simulink model "DatcomNew"  (R2017a)
settings: Solver=VariableStepAuto  StartTime=0.0  StopTime=10.0  RelTol=1e-3
undefined symbols (not defined in the file or in its folder): datcom, Newton, Raphson
libraries: aerolibutil x32, sharedutil x4, aerolibtransform2 x3, aerolibasang x3, aerolibadyn x1
(part 2 of 4)

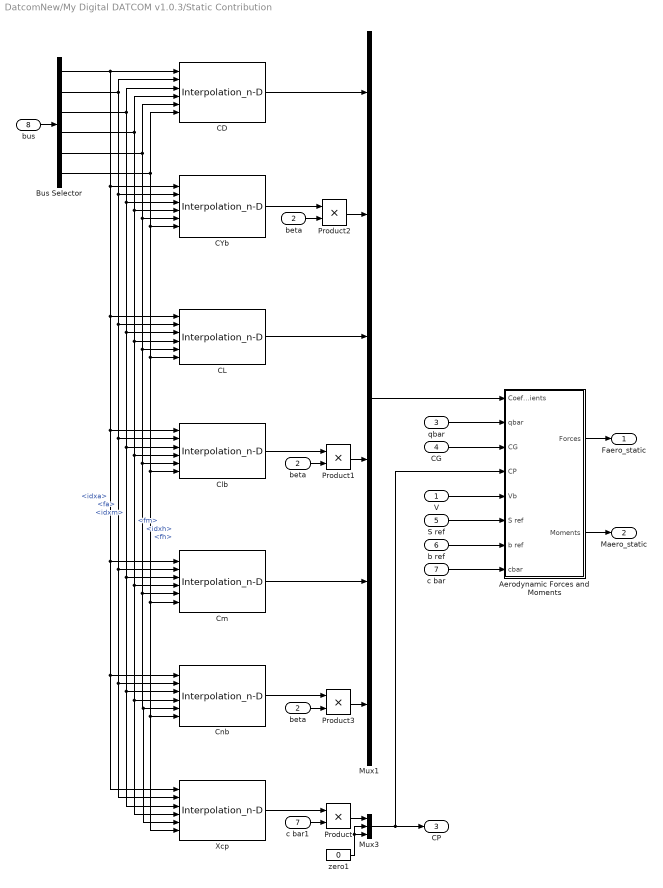
== system DatcomNew/My Digital DATCOM v1.0.3/Static Contribution ==
  "V " : Inport
  beta : Inport  Port=2
  qbar : Inport  Port=3
  CG : Inport  Port=4
  S ref : Inport  Port=5  Unit=m^2
  b ref : Inport  Port=6  Unit=m  PortDimensions=1
  c bar : Inport  Port=7  Unit=m  PortDimensions=1
  bus : Inport  Port=8
  " beta " : InportShadow  Port=2
  Aerodynamic Forces and Moments : Subsystem
  Bus Selector : BusSelector  OutputSignals=idxa,fa,idxm,fm,idxh,fh
  CD : Interpolation_n-D  NumberOfTableDimensions=3  Table=permute(datcom.cd,[1 2 3])  InterpMethod=Flat  ExtrapMethod=Clip  OutDataTypeStr=double
      settings: InputPortMap=u0,u1,u2,u3,u4,u5
  CL : Interpolation_n-D  NumberOfTableDimensions=3  Table=permute(datcom.cl,[1 2 3])  InterpMethod=Flat  ExtrapMethod=Clip  OutDataTypeStr=double
      settings: InputPortMap=u0,u1,u2,u3,u4,u5
  CYb : Interpolation_n-D  NumberOfTableDimensions=3  Table=permute(datcom.cyb,[1 2 3])  InterpMethod=Flat  ExtrapMethod=Clip  OutDataTypeStr=double
      settings: InputPortMap=u0,u1,u2,u3,u4,u5
  Clb : Interpolation_n-D  NumberOfTableDimensions=3  Table=permute(datcom.clb,[1 2 3])  InterpMethod=Flat  ExtrapMethod=Clip  OutDataTypeStr=double
      settings: InputPortMap=u0,u1,u2,u3,u4,u5
  Cm : Interpolation_n-D  NumberOfTableDimensions=3  Table=permute(datcom.cm,[1 2 3])  InterpMethod=Flat  ExtrapMethod=Clip  OutDataTypeStr=double
      settings: InputPortMap=u0,u1,u2,u3,u4,u5
  Cnb : Interpolation_n-D  NumberOfTableDimensions=3  Table=permute(datcom.cnb,[1 2 3])  InterpMethod=Flat  ExtrapMethod=Clip  OutDataTypeStr=double
      settings: InputPortMap=u0,u1,u2,u3,u4,u5
  Mux1 : Mux  Inputs=6
  Mux3 : Mux  Inputs=3
  Product : Product
  Product1 : Product  RndMeth=Zero
  Product2 : Product  RndMeth=Zero
  Product3 : Product  RndMeth=Zero
  Xcp : Interpolation_n-D  NumberOfTableDimensions=3  Table="permute(datcom.xcp,[1  2  3])"  OutDataTypeStr=double
      settings: InputPortMap=u0,u1,u2,u3,u4,u5
  "beta " : InportShadow  Port=2
  c bar1 : InportShadow  Port=7  Unit=m  PortDimensions=1
  zero1 : Constant  Value=0
  Faero_static : Outport
  Maero_static : Outport  Port=2
  "CP " : Outport  Port=3
  wires:
  c bar1/1 -> Product/2
  Product/1 -> Mux3/1
  zero1/1 -> Mux3/3, Mux3/2
  Xcp/1 -> Product/1
  c bar/1 -> Aerodynamic Forces and Moments/8(cbar)
  b ref/1 -> Aerodynamic Forces and Moments/7(b ref)
  S ref/1 -> Aerodynamic Forces and Moments/6(S ref)
  Mux3/1 -> Aerodynamic Forces and Moments/4(CP), "CP "/1
  CG/1 -> Aerodynamic Forces and Moments/3(CG)
  bus/1 -> Bus Selector/1
  Bus Selector/1 -> CD/1, CYb/1, Clb/1, Cnb/1, Xcp/1, Cm/1, CL/1  "<idxa>"
  Bus Selector/2 -> Cnb/2, Xcp/2, Cm/2, Clb/2, CL/2, CYb/2, CD/2  "<fa>"
  Bus Selector/3 -> Cnb/3, Xcp/3, Cm/3, Clb/3, CL/3, CYb/3, CD/3  "<idxm>"
  Bus Selector/4 -> Cnb/4, Xcp/4, Cm/4, Clb/4, CL/4, CYb/4, CD/4  "<fm>"
  Bus Selector/5 -> Cnb/5, Xcp/5, Cm/5, Clb/5, CL/5, CYb/5, CD/5  "<idxh>"
  Bus Selector/6 -> Cnb/6, Xcp/6, Cm/6, Clb/6, CL/6, CYb/6, CD/6  "<fh>"
  CD/1 -> Mux1/1
  CL/1 -> Mux1/3
  CYb/1 -> Product2/1
  beta/1 -> Product2/2
  Clb/1 -> Product1/1
  "beta "/1 -> Product1/2
  Product2/1 -> Mux1/2
  Product1/1 -> Mux1/4
  Cm/1 -> Mux1/5
  Cnb/1 -> Product3/1
  " beta "/1 -> Product3/2
  Product3/1 -> Mux1/6
  Mux1/1 -> Aerodynamic Forces and Moments/1(Coefficients)
  Aerodynamic Forces and Moments/1(Forces) -> Faero_static/1
  qbar/1 -> Aerodynamic Forces and Moments/2(qbar)
  Aerodynamic Forces and Moments/2(Moments) -> Maero_static/1
  "V "/1 -> Aerodynamic Forces and Moments/5(Vb)

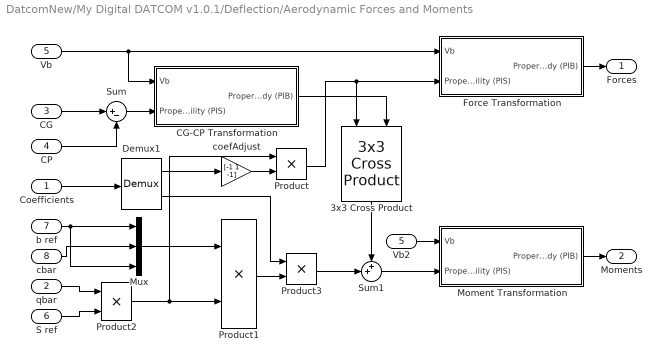
== system DatcomNew/My Digital DATCOM v1.0.1/Deflection/Aerodynamic Forces and Moments ==
  Coefficients : Inport
  qbar : Inport  Port=2  Unit=Pa
  CG : Inport  Port=3  Unit=m  PortDimensions=[3, 1]
  CP : Inport  Port=4  Unit=m  PortDimensions=[3,1]
  Vb : Inport  Port=5
  S ref : Inport  Port=6  Unit=m^2  PortDimensions=1
  b ref : Inport  Port=7  Unit=m  PortDimensions=1
  cbar : Inport  Port=8  Unit=m  PortDimensions=1
  3x3 Cross Product : aerolibutil/3x3 Cross Product
      settings: SourceProductName=Aerospace Blockset  SourceProductBaseCode=AE
  CG-CP Transformation : Subsystem
  Demux1 : Demux  Outputs=[3,3]
  Force Transformation : Subsystem
  Moment Transformation : Subsystem
  Mux : Mux  Inputs=3
  Product{,1..3} (4 alike) : Product  SaturateOnIntegerOverflow=on  InputSameDT=on  OutDataTypeStr=Inherit: Same as first input
  Sum : Sum  Inputs=|+-  SaturateOnIntegerOverflow=on
  Sum1 : Sum  Inputs=++|  SaturateOnIntegerOverflow=on  InputSameDT=on  OutDataTypeStr=Inherit: Same as first input
  Vb2 : InportShadow  Port=5
  coefAdjust : Gain  Gain="[-1  1 -1]"
  Forces : Outport  Unit=N
  Moments : Outport  Port=2  Unit=N
  wires:
  Vb/1 -> CG-CP Transformation/1(Vb), Force Transformation/1(Vb)
  CG-CP Transformation/1(Property-In-Body (PIB)) -> 3x3 Cross Product/2
  Sum/1 -> CG-CP Transformation/2(Property-In-Stability (PIS))
  CP/1 -> Sum/2
  CG/1 -> Sum/1
  coefAdjust/1 -> Product/2
  Moment Transformation/1(Property-In-Body (PIB)) -> Moments/1
  Force Transformation/1(Property-In-Body (PIB)) -> Forces/1
  Product/1 -> 3x3 Cross Product/1, Force Transformation/2(Property-In-Stability (PIS))
  Demux1/1 -> coefAdjust/1
  Product3/1 -> Sum1/2
  Product2/1 -> Product/1, Product1/2
  qbar/1 -> Product2/1
  Demux1/2 -> Product3/1
  Coefficients/1 -> Demux1/1
  Product1/1 -> Product3/2
  3x3 Cross Product/1 -> Sum1/1
  cbar/1 -> Mux/2
  b ref/1 -> Mux/1, Mux/3
  Mux/1 -> Product1/1
  S ref/1 -> Product2/2
  Sum1/1 -> Moment Transformation/2(Property-In-Stability (PIS))
  Vb2/1 -> Moment Transformation/1(Vb)

== system DatcomNew/My Digital DATCOM v1.0.1/Deflection/Delta Coefficients ==
  bus : Inport
  Aileron Deflaction : Subsystem
  Elevator Deflaction : Subsystem
  Flap Deflaction : Subsystem
  Sum : Sum  Inputs=+++
  delCoeff : Outport
  wires:
  bus/1 -> Flap Deflaction/1(bus), Aileron Deflaction/1(bus), Elevator Deflaction/1(bus)
  Elevator Deflaction/1(delCoeff_e) -> Sum/2
  Flap Deflaction/1(delCoeff_f) -> Sum/1
  Aileron Deflaction/1(delCoeff_a) -> Sum/3
  Sum/1 -> delCoeff/1

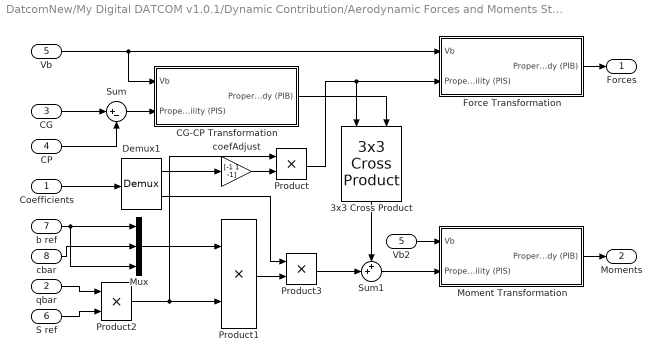
== system DatcomNew/My Digital DATCOM v1.0.1/Dynamic Contribution/Aerodynamic Forces and Moments Stability Axis ==
  Coefficients : Inport
  qbar : Inport  Port=2  Unit=Pa
  CG : Inport  Port=3  Unit=m  PortDimensions=[3, 1]
  CP : Inport  Port=4  Unit=m  PortDimensions=[3,1]
  Vb : Inport  Port=5
  S ref : Inport  Port=6  Unit=m^2  PortDimensions=1
  b ref : Inport  Port=7  Unit=m  PortDimensions=1
  cbar : Inport  Port=8  Unit=m  PortDimensions=1
  3x3 Cross Product : aerolibutil/3x3 Cross Product
      settings: SourceProductName=Aerospace Blockset  SourceProductBaseCode=AE
  CG-CP Transformation : Subsystem
  Demux1 : Demux  Outputs=[3,3]
  Force Transformation : Subsystem
  Moment Transformation : Subsystem
  Mux : Mux  Inputs=3
  Product{,1..3} (4 alike) : Product  SaturateOnIntegerOverflow=on  InputSameDT=on  OutDataTypeStr=Inherit: Same as first input
  Sum : Sum  Inputs=|+-  SaturateOnIntegerOverflow=on
  Sum1 : Sum  Inputs=++|  SaturateOnIntegerOverflow=on  InputSameDT=on  OutDataTypeStr=Inherit: Same as first input
  Vb2 : InportShadow  Port=5
  coefAdjust : Gain  Gain="[-1  1 -1]"
  Forces : Outport  Unit=N
  Moments : Outport  Port=2  Unit=N*m
  wires:
  Vb/1 -> CG-CP Transformation/1(Vb), Force Transformation/1(Vb)
  CG-CP Transformation/1(Property-In-Body (PIB)) -> 3x3 Cross Product/2
  Sum/1 -> CG-CP Transformation/2(Property-In-Stability (PIS))
  CP/1 -> Sum/2
  CG/1 -> Sum/1
  coefAdjust/1 -> Product/2
  Moment Transformation/1(Property-In-Body (PIB)) -> Moments/1
  Force Transformation/1(Property-In-Body (PIB)) -> Forces/1
  Product/1 -> 3x3 Cross Product/1, Force Transformation/2(Property-In-Stability (PIS))
  Demux1/1 -> coefAdjust/1
  Product3/1 -> Sum1/2
  Product2/1 -> Product/1, Product1/2
  qbar/1 -> Product2/1
  Demux1/2 -> Product3/1
  Coefficients/1 -> Demux1/1
  Product1/1 -> Product3/2
  3x3 Cross Product/1 -> Sum1/1
  cbar/1 -> Mux/2
  b ref/1 -> Mux/1, Mux/3
  Mux/1 -> Product1/1
  S ref/1 -> Product2/2
  Sum1/1 -> Moment Transformation/2(Property-In-Stability (PIS))
  Vb2/1 -> Moment Transformation/1(Vb)

== system DatcomNew/My Digital DATCOM v1.0.1/Dynamic Contribution/Incidence, Sideslip, & Airspeed1 ==
  Vb : Inport  Unit=m/s
  Airspeed : Sqrt  AlgorithmType=Newton-Raphson  SaturateOnIntegerOverflow=on
  Dot Product : DotProduct  InputSameDT=on  OutDataTypeStr=Inherit: Inherit via internal rule
  Incidence : Trigonometry  Operator=atan2
  Product : Product  Inputs=*/  SaturateOnIntegerOverflow=on  OutDataTypeStr=Inherit: Same as first input
  Selector : Selector  InputPortWidth=3  IndexOptions=Index vector (dialog)  Indices=[2]  OutputSizes=1
  Selector1 : Selector  InputPortWidth=3  IndexOptions=Index vector (dialog)  Indices=[3]  OutputSizes=1
  Selector2 : Selector  InputPortWidth=3  IndexOptions=Index vector (dialog)  Indices=[1]  OutputSizes=1
  Sideslip : Trigonometry  Operator=asin
  Alpha : Outport  Unit=rad  InitialOutput=0
  Beta : Outport  Port=2  Unit=rad  InitialOutput=0
  V : Outport  Port=3  Unit=m/s  InitialOutput=0
  wires:
  Product/1 -> Sideslip/1
  Selector1/1 -> Incidence/1
  Selector2/1 -> Incidence/2
  Dot Product/1 -> Airspeed/1
  Airspeed/1 -> Product/2, V/1
  Incidence/1 -> Alpha/1
  Vb/1 -> Selector1/1, Selector2/1, Selector/1, Dot Product/1, Dot Product/2
  Sideslip/1 -> Beta/1
  Selector/1 -> Product/1

== system DatcomNew/My Digital DATCOM v1.0.1/Dynamic Contribution/Stability Angular Rates ==
  alpha beta : Inport  Unit=rad
  alphadot betadot : Inport  Port=2  Unit=rad/s
  p,q,r : Inport  Port=3  Unit=rad/s
  Demux : Demux  Outputs=2
  Direction Cosine Matrix Body to Wind : aerolibtransform2/Direction Cosine Matrix Body to Wind
      settings: SourceProductName=Aerospace Blockset  SourceProductBaseCode=AE
  Disallow CGS : UnitConfiguration  UnitSystemsStr=English,SI,SI (extended)  AllowAllUnitSystems=off
  Mux : Mux  Inputs=3
  Product : Product  RndMeth=Zero
  Product1 : Product  Multiplication=Matrix(*)  SaturateOnIntegerOverflow=on  InputSameDT=on  OutDataTypeStr=Inherit: Same as first input
  Product2 : Product  RndMeth=Zero
  SinCos : Trigonometry  Operator=sincos
  Subsystem : aerolibasang/Wind Angular Rates/Subsystem
      settings: SourceProductName=Aerospace Blockset  SourceProductBaseCode=AE
  Sum : Sum  Inputs=|++
  Unary Minus : UnaryMinus
  Unary Minus1 : UnaryMinus
  p,q,r wind : Outport  Unit=rad/s  InitialOutput=0
  wires:
  Unary Minus/1 -> Mux/2
  Unary Minus1/1 -> Mux/1
  Product2/1 -> Mux/3
  Product/1 -> Unary Minus1/1
  Demux/1 -> Unary Minus/1
  Demux/2 -> Product/1, Product2/1
  alphadot betadot/1 -> Demux/1
  p,q,r/1 -> Sum/2
  Mux/1 -> Sum/1
  Product1/1 -> p,q,r wind/1
  Sum/1 -> Product1/2
  Direction Cosine Matrix Body to Wind/1 -> Product1/1
  SinCos/2 -> Product2/2
  SinCos/1 -> Product/2
  Subsystem/1 -> SinCos/1
  alpha beta/1 -> Subsystem/1, Direction Cosine Matrix Body to Wind/1

== system DatcomNew/My Digital DATCOM v1.0.1/Static Contribution/Aerodynamic Forces and Moments ==
  Coefficients : Inport
  qbar : Inport  Port=2  Unit=Pa
  CG : Inport  Port=3  Unit=m  PortDimensions=[3, 1]
  CP : Inport  Port=4  Unit=m  PortDimensions=[3,1]
  Vb : Inport  Port=5
  S ref : Inport  Port=6  Unit=m^2  PortDimensions=1
  b ref : Inport  Port=7  Unit=m  PortDimensions=1
  cbar : Inport  Port=8  Unit=m  PortDimensions=1
  3x3 Cross Product : aerolibutil/3x3 Cross Product
      settings: SourceProductName=Aerospace Blockset  SourceProductBaseCode=AE
  CG-CP Transformation : Subsystem
  Demux1 : Demux  Outputs=[3,3]
  Force Transformation : Subsystem
  Moment Transformation : Subsystem
  Mux : Mux  Inputs=3
  Product{,1..3} (4 alike) : Product  SaturateOnIntegerOverflow=on  InputSameDT=on  OutDataTypeStr=Inherit: Same as first input
  Sum : Sum  Inputs=|+-  SaturateOnIntegerOverflow=on
  Sum1 : Sum  Inputs=++|  SaturateOnIntegerOverflow=on  InputSameDT=on  OutDataTypeStr=Inherit: Same as first input
  Vb2 : InportShadow  Port=5
  coefAdjust : Gain  Gain="[-1  1 -1]"
  Forces : Outport  Unit=N
  Moments : Outport  Port=2  Unit=N*m
  wires:
  Vb/1 -> CG-CP Transformation/1(Vb), Force Transformation/1(Vb)
  CG-CP Transformation/1(Property-In-Body (PIB)) -> 3x3 Cross Product/2
  Sum/1 -> CG-CP Transformation/2(Property-In-Stability (PIS))
  CP/1 -> Sum/2
  CG/1 -> Sum/1
  coefAdjust/1 -> Product/2
  Moment Transformation/1(Property-In-Body (PIB)) -> Moments/1
  Force Transformation/1(Property-In-Body (PIB)) -> Forces/1
  Product/1 -> 3x3 Cross Product/1, Force Transformation/2(Property-In-Stability (PIS))
  Demux1/1 -> coefAdjust/1
  Product3/1 -> Sum1/2
  Product2/1 -> Product/1, Product1/2
  qbar/1 -> Product2/1
  Demux1/2 -> Product3/1
  Coefficients/1 -> Demux1/1
  Product1/1 -> Product3/2
  3x3 Cross Product/1 -> Sum1/1
  cbar/1 -> Mux/2
  b ref/1 -> Mux/1, Mux/3
  Mux/1 -> Product1/1
  S ref/1 -> Product2/2
  Sum1/1 -> Moment Transformation/2(Property-In-Stability (PIS))
  Vb2/1 -> Moment Transformation/1(Vb)

== system DatcomNew/My Digital DATCOM v1.0.2/Deflection/Aerodynamic Forces and Moments ==
  Coefficients : Inport
  qbar : Inport  Port=2  Unit=Pa
  CG : Inport  Port=3  Unit=m  PortDimensions=[3, 1]
  CP : Inport  Port=4  Unit=m  PortDimensions=[3,1]
  Vb : Inport  Port=5
  S ref : Inport  Port=6  Unit=m^2  PortDimensions=1
  b ref : Inport  Port=7  Unit=m  PortDimensions=1
  cbar : Inport  Port=8  Unit=m  PortDimensions=1
  3x3 Cross Product : aerolibutil/3x3 Cross Product
      settings: SourceProductName=Aerospace Blockset  SourceProductBaseCode=AE
  CG-CP Transformation : Subsystem
  Demux1 : Demux  Outputs=[3,3]
  Force Transformation : Subsystem
  Moment Transformation : Subsystem
  Mux : Mux  Inputs=3
  Product{,1..3} (4 alike) : Product  SaturateOnIntegerOverflow=on  InputSameDT=on  OutDataTypeStr=Inherit: Same as first input
  Sum : Sum  Inputs=|+-  SaturateOnIntegerOverflow=on
  Sum1 : Sum  Inputs=++|  SaturateOnIntegerOverflow=on  InputSameDT=on  OutDataTypeStr=Inherit: Same as first input
  Vb2 : InportShadow  Port=5
  coefAdjust : Gain  Gain="[-1  1 -1]"
  Forces : Outport  Unit=N
  Moments : Outport  Port=2  Unit=N
  wires:
  Vb2/1 -> Moment Transformation/1(Vb)
  Sum1/1 -> Moment Transformation/2(Property-In-Stability (PIS))
  S ref/1 -> Product2/2
  Mux/1 -> Product1/1
  b ref/1 -> Mux/3, Mux/1
  cbar/1 -> Mux/2
  3x3 Cross Product/1 -> Sum1/1
  Product1/1 -> Product3/2
  Coefficients/1 -> Demux1/1
  Demux1/2 -> Product3/1
  qbar/1 -> Product2/1
  Product2/1 -> Product1/2, Product/1
  Product3/1 -> Sum1/2
  Demux1/1 -> coefAdjust/1
  Product/1 -> Force Transformation/2(Property-In-Stability (PIS)), 3x3 Cross Product/1
  Force Transformation/1(Property-In-Body (PIB)) -> Forces/1
  Moment Transformation/1(Property-In-Body (PIB)) -> Moments/1
  coefAdjust/1 -> Product/2
  CG/1 -> Sum/1
  CP/1 -> Sum/2
  Sum/1 -> CG-CP Transformation/2(Property-In-Stability (PIS))
  CG-CP Transformation/1(Property-In-Body (PIB)) -> 3x3 Cross Product/2
  Vb/1 -> Force Transformation/1(Vb), CG-CP Transformation/1(Vb)

== system DatcomNew/My Digital DATCOM v1.0.2/Deflection/Delta Coefficients ==
  bus : Inport
  Aileron Deflaction : Subsystem
  Elevator Deflaction : Subsystem
  Flap Deflaction : Subsystem
  Sum : Sum  Inputs=+++
  delCoeff : Outport
  wires:
  Sum/1 -> delCoeff/1
  Aileron Deflaction/1(delCoeff_a) -> Sum/3
  Flap Deflaction/1(delCoeff_f) -> Sum/1
  Elevator Deflaction/1(delCoeff_e) -> Sum/2
  bus/1 -> Elevator Deflaction/1(bus), Aileron Deflaction/1(bus), Flap Deflaction/1(bus)

== system DatcomNew/My Digital DATCOM v1.0.2/Dynamic Contribution/Aerodynamic Forces and Moments Stability Axis ==
  Coefficients : Inport
  qbar : Inport  Port=2  Unit=Pa
  CG : Inport  Port=3  Unit=m  PortDimensions=[3, 1]
  CP : Inport  Port=4  Unit=m  PortDimensions=[3,1]
  Vb : Inport  Port=5
  S ref : Inport  Port=6  Unit=m^2  PortDimensions=1
  b ref : Inport  Port=7  Unit=m  PortDimensions=1
  cbar : Inport  Port=8  Unit=m  PortDimensions=1
  3x3 Cross Product : aerolibutil/3x3 Cross Product
      settings: SourceProductName=Aerospace Blockset  SourceProductBaseCode=AE
  CG-CP Transformation : Subsystem
  Demux1 : Demux  Outputs=[3,3]
  Force Transformation : Subsystem
  Moment Transformation : Subsystem
  Mux : Mux  Inputs=3
  Product{,1..3} (4 alike) : Product  SaturateOnIntegerOverflow=on  InputSameDT=on  OutDataTypeStr=Inherit: Same as first input
  Sum : Sum  Inputs=|+-  SaturateOnIntegerOverflow=on
  Sum1 : Sum  Inputs=++|  SaturateOnIntegerOverflow=on  InputSameDT=on  OutDataTypeStr=Inherit: Same as first input
  Vb2 : InportShadow  Port=5
  coefAdjust : Gain  Gain="[-1  1 -1]"
  Forces : Outport  Unit=N
  Moments : Outport  Port=2  Unit=N*m
  wires:
  Vb2/1 -> Moment Transformation/1(Vb)
  Sum1/1 -> Moment Transformation/2(Property-In-Stability (PIS))
  S ref/1 -> Product2/2
  Mux/1 -> Product1/1
  b ref/1 -> Mux/3, Mux/1
  cbar/1 -> Mux/2
  3x3 Cross Product/1 -> Sum1/1
  Product1/1 -> Product3/2
  Coefficients/1 -> Demux1/1
  Demux1/2 -> Product3/1
  qbar/1 -> Product2/1
  Product2/1 -> Product1/2, Product/1
  Product3/1 -> Sum1/2
  Demux1/1 -> coefAdjust/1
  Product/1 -> Force Transformation/2(Property-In-Stability (PIS)), 3x3 Cross Product/1
  Force Transformation/1(Property-In-Body (PIB)) -> Forces/1
  Moment Transformation/1(Property-In-Body (PIB)) -> Moments/1
  coefAdjust/1 -> Product/2
  CG/1 -> Sum/1
  CP/1 -> Sum/2
  Sum/1 -> CG-CP Transformation/2(Property-In-Stability (PIS))
  CG-CP Transformation/1(Property-In-Body (PIB)) -> 3x3 Cross Product/2
  Vb/1 -> Force Transformation/1(Vb), CG-CP Transformation/1(Vb)

== system DatcomNew/My Digital DATCOM v1.0.2/Dynamic Contribution/Incidence, Sideslip, & Airspeed1 ==
  Vb : Inport  Unit=m/s
  Airspeed : Sqrt  AlgorithmType=Newton-Raphson  SaturateOnIntegerOverflow=on
  Dot Product : DotProduct  InputSameDT=on  OutDataTypeStr=Inherit: Inherit via internal rule
  Incidence : Trigonometry  Operator=atan2
  Product : Product  Inputs=*/  SaturateOnIntegerOverflow=on  OutDataTypeStr=Inherit: Same as first input
  Selector : Selector  InputPortWidth=3  IndexOptions=Index vector (dialog)  Indices=[2]  OutputSizes=1
  Selector1 : Selector  InputPortWidth=3  IndexOptions=Index vector (dialog)  Indices=[3]  OutputSizes=1
  Selector2 : Selector  InputPortWidth=3  IndexOptions=Index vector (dialog)  Indices=[1]  OutputSizes=1
  Sideslip : Trigonometry  Operator=asin
  Alpha : Outport  Unit=rad  InitialOutput=0
  Beta : Outport  Port=2  Unit=rad  InitialOutput=0
  V : Outport  Port=3  Unit=m/s  InitialOutput=0
  wires:
  Selector/1 -> Product/1
  Sideslip/1 -> Beta/1
  Vb/1 -> Dot Product/2, Dot Product/1, Selector/1, Selector2/1, Selector1/1
  Incidence/1 -> Alpha/1
  Airspeed/1 -> V/1, Product/2
  Dot Product/1 -> Airspeed/1
  Selector2/1 -> Incidence/2
  Selector1/1 -> Incidence/1
  Product/1 -> Sideslip/1

== system DatcomNew/My Digital DATCOM v1.0.2/Dynamic Contribution/Stability Angular Rates ==
  alpha beta : Inport  Unit=rad
  alphadot betadot : Inport  Port=2  Unit=rad/s
  p,q,r : Inport  Port=3  Unit=rad/s
  Demux : Demux  Outputs=2
  Direction Cosine Matrix Body to Wind : aerolibtransform2/Direction Cosine Matrix Body to Wind
      settings: SourceProductName=Aerospace Blockset  SourceProductBaseCode=AE
  Disallow CGS : UnitConfiguration  UnitSystemsStr=English,SI,SI (extended)  AllowAllUnitSystems=off
  Mux : Mux  Inputs=3
  Product : Product  RndMeth=Zero
  Product1 : Product  Multiplication=Matrix(*)  SaturateOnIntegerOverflow=on  InputSameDT=on  OutDataTypeStr=Inherit: Same as first input
  Product2 : Product  RndMeth=Zero
  SinCos : Trigonometry  Operator=sincos
  Subsystem : aerolibasang/Wind Angular Rates/Subsystem
      settings: SourceProductName=Aerospace Blockset  SourceProductBaseCode=AE
  Sum : Sum  Inputs=|++
  Unary Minus : UnaryMinus
  Unary Minus1 : UnaryMinus
  p,q,r wind : Outport  Unit=rad/s  InitialOutput=0
  wires:
  alpha beta/1 -> Direction Cosine Matrix Body to Wind/1, Subsystem/1
  Subsystem/1 -> SinCos/1
  SinCos/1 -> Product/2
  SinCos/2 -> Product2/2
  Direction Cosine Matrix Body to Wind/1 -> Product1/1
  Sum/1 -> Product1/2
  Product1/1 -> p,q,r wind/1
  Mux/1 -> Sum/1
  p,q,r/1 -> Sum/2
  alphadot betadot/1 -> Demux/1
  Demux/2 -> Product2/1, Product/1
  Demux/1 -> Unary Minus/1
  Product/1 -> Unary Minus1/1
  Product2/1 -> Mux/3
  Unary Minus1/1 -> Mux/1
  Unary Minus/1 -> Mux/2

== system DatcomNew/My Digital DATCOM v1.0.2/Static Contribution/Aerodynamic Forces and Moments ==
  Coefficients : Inport
  qbar : Inport  Port=2  Unit=Pa
  CG : Inport  Port=3  Unit=m  PortDimensions=[3, 1]
  CP : Inport  Port=4  Unit=m  PortDimensions=[3,1]
  Vb : Inport  Port=5
  S ref : Inport  Port=6  Unit=m^2  PortDimensions=1
  b ref : Inport  Port=7  Unit=m  PortDimensions=1
  cbar : Inport  Port=8  Unit=m  PortDimensions=1
  3x3 Cross Product : aerolibutil/3x3 Cross Product
      settings: SourceProductName=Aerospace Blockset  SourceProductBaseCode=AE
  CG-CP Transformation : Subsystem
  Demux1 : Demux  Outputs=[3,3]
  Force Transformation : Subsystem
  Moment Transformation : Subsystem
  Mux : Mux  Inputs=3
  Product{,1..3} (4 alike) : Product  SaturateOnIntegerOverflow=on  InputSameDT=on  OutDataTypeStr=Inherit: Same as first input
  Sum : Sum  Inputs=|+-  SaturateOnIntegerOverflow=on
  Sum1 : Sum  Inputs=++|  SaturateOnIntegerOverflow=on  InputSameDT=on  OutDataTypeStr=Inherit: Same as first input
  Vb2 : InportShadow  Port=5
  coefAdjust : Gain  Gain="[-1  1 -1]"
  Forces : Outport  Unit=N
  Moments : Outport  Port=2  Unit=N*m
  wires:
  Vb2/1 -> Moment Transformation/1(Vb)
  Sum1/1 -> Moment Transformation/2(Property-In-Stability (PIS))
  S ref/1 -> Product2/2
  Mux/1 -> Product1/1
  b ref/1 -> Mux/3, Mux/1
  cbar/1 -> Mux/2
  3x3 Cross Product/1 -> Sum1/1
  Product1/1 -> Product3/2
  Coefficients/1 -> Demux1/1
  Demux1/2 -> Product3/1
  qbar/1 -> Product2/1
  Product2/1 -> Product1/2, Product/1
  Product3/1 -> Sum1/2
  Demux1/1 -> coefAdjust/1
  Product/1 -> Force Transformation/2(Property-In-Stability (PIS)), 3x3 Cross Product/1
  Force Transformation/1(Property-In-Body (PIB)) -> Forces/1
  Moment Transformation/1(Property-In-Body (PIB)) -> Moments/1
  coefAdjust/1 -> Product/2
  CG/1 -> Sum/1
  CP/1 -> Sum/2
  Sum/1 -> CG-CP Transformation/2(Property-In-Stability (PIS))
  CG-CP Transformation/1(Property-In-Body (PIB)) -> 3x3 Cross Product/2
  Vb/1 -> Force Transformation/1(Vb), CG-CP Transformation/1(Vb)

== system DatcomNew/My Digital DATCOM v1.0.3/Deflection/Aerodynamic Forces and Moments ==
  Coefficients : Inport
  qbar : Inport  Port=2  Unit=Pa
  CG : Inport  Port=3  Unit=m  PortDimensions=[3, 1]
  CP : Inport  Port=4  Unit=m  PortDimensions=[3,1]
  Vb : Inport  Port=5
  S ref : Inport  Port=6  Unit=m^2  PortDimensions=1
  b ref : Inport  Port=7  Unit=m  PortDimensions=1
  cbar : Inport  Port=8  Unit=m  PortDimensions=1
  3x3 Cross Product : aerolibutil/3x3 Cross Product
      settings: SourceProductName=Aerospace Blockset  SourceProductBaseCode=AE
  CG-CP Transformation : Subsystem
  Demux1 : Demux  Outputs=[3,3]
  Force Transformation : Subsystem
  Moment Transformation : Subsystem
  Mux : Mux  Inputs=3
  Product{,1..3} (4 alike) : Product  SaturateOnIntegerOverflow=on  InputSameDT=on  OutDataTypeStr=Inherit: Same as first input
  Sum : Sum  Inputs=|+-  SaturateOnIntegerOverflow=on
  Sum1 : Sum  Inputs=++|  SaturateOnIntegerOverflow=on  InputSameDT=on  OutDataTypeStr=Inherit: Same as first input
  Vb2 : InportShadow  Port=5
  coefAdjust : Gain  Gain="[-1  1 -1]"
  Forces : Outport  Unit=N
  Moments : Outport  Port=2  Unit=N
  wires:
  Vb2/1 -> Moment Transformation/1(Vb)
  Sum1/1 -> Moment Transformation/2(Property-In-Stability (PIS))
  S ref/1 -> Product2/2
  Mux/1 -> Product1/1
  b ref/1 -> Mux/3, Mux/1
  cbar/1 -> Mux/2
  3x3 Cross Product/1 -> Sum1/1
  Product1/1 -> Product3/2
  Coefficients/1 -> Demux1/1
  Demux1/2 -> Product3/1
  qbar/1 -> Product2/1
  Product2/1 -> Product1/2, Product/1
  Product3/1 -> Sum1/2
  Demux1/1 -> coefAdjust/1
  Product/1 -> Force Transformation/2(Property-In-Stability (PIS)), 3x3 Cross Product/1
  Force Transformation/1(Property-In-Body (PIB)) -> Forces/1
  Moment Transformation/1(Property-In-Body (PIB)) -> Moments/1
  coefAdjust/1 -> Product/2
  CG/1 -> Sum/1
  CP/1 -> Sum/2
  Sum/1 -> CG-CP Transformation/2(Property-In-Stability (PIS))
  CG-CP Transformation/1(Property-In-Body (PIB)) -> 3x3 Cross Product/2
  Vb/1 -> Force Transformation/1(Vb), CG-CP Transformation/1(Vb)

== system DatcomNew/My Digital DATCOM v1.0.3/Deflection/Delta Coefficients ==
  bus : Inport
  Aileron Deflaction : Subsystem
  Elevator Deflaction : Subsystem
  Flap Deflaction : Subsystem
  Sum : Sum  Inputs=+++
  delCoeff : Outport
  wires:
  Sum/1 -> delCoeff/1
  Aileron Deflaction/1(delCoeff_a) -> Sum/3
  Flap Deflaction/1(delCoeff_f) -> Sum/1
  Elevator Deflaction/1(delCoeff_e) -> Sum/2
  bus/1 -> Elevator Deflaction/1(bus), Aileron Deflaction/1(bus), Flap Deflaction/1(bus)

== system DatcomNew/My Digital DATCOM v1.0.3/Dynamic Contribution/Aerodynamic Forces and Moments Stability Axis ==
  Coefficients : Inport
  qbar : Inport  Port=2  Unit=Pa
  CG : Inport  Port=3  Unit=m  PortDimensions=[3, 1]
  CP : Inport  Port=4  Unit=m  PortDimensions=[3,1]
  Vb : Inport  Port=5
  S ref : Inport  Port=6  Unit=m^2  PortDimensions=1
  b ref : Inport  Port=7  Unit=m  PortDimensions=1
  cbar : Inport  Port=8  Unit=m  PortDimensions=1
  3x3 Cross Product : sharedutil/3x3 Cross Product
  CG-CP Transformation : Subsystem
  Demux1 : Demux  Outputs=[3,3]
  Force Transformation : Subsystem
  Moment Transformation : Subsystem
  Mux : Mux  Inputs=3
  Product{,1..3} (4 alike) : Product  SaturateOnIntegerOverflow=on  InputSameDT=on  OutDataTypeStr=Inherit: Same as first input
  Sum : Sum  Inputs=|+-  SaturateOnIntegerOverflow=on
  Sum1 : Sum  Inputs=++|  SaturateOnIntegerOverflow=on  InputSameDT=on  OutDataTypeStr=Inherit: Same as first input
  Vb2 : InportShadow  Port=5
  coefAdjust : Gain  Gain="[-1  1 -1]"
  Forces : Outport  Unit=N
  Moments : Outport  Port=2  Unit=N*m
  wires:
  Vb2/1 -> Moment Transformation/1(Vb)
  Sum1/1 -> Moment Transformation/2(Property-In-Stability (PIS))
  S ref/1 -> Product2/2
  Mux/1 -> Product1/1
  b ref/1 -> Mux/3, Mux/1
  cbar/1 -> Mux/2
  3x3 Cross Product/1 -> Sum1/1
  Product1/1 -> Product3/2
  Coefficients/1 -> Demux1/1
  Demux1/2 -> Product3/1
  qbar/1 -> Product2/1
  Product2/1 -> Product1/2, Product/1
  Product3/1 -> Sum1/2
  Demux1/1 -> coefAdjust/1
  Product/1 -> Force Transformation/2(Property-In-Stability (PIS)), 3x3 Cross Product/1
  Force Transformation/1(Property-In-Body (PIB)) -> Forces/1
  Moment Transformation/1(Property-In-Body (PIB)) -> Moments/1
  coefAdjust/1 -> Product/2
  CG/1 -> Sum/1
  CP/1 -> Sum/2
  Sum/1 -> CG-CP Transformation/2(Property-In-Stability (PIS))
  CG-CP Transformation/1(Property-In-Body (PIB)) -> 3x3 Cross Product/2
  Vb/1 -> Force Transformation/1(Vb), CG-CP Transformation/1(Vb)

== system DatcomNew/My Digital DATCOM v1.0.3/Dynamic Contribution/Incidence, Sideslip, & Airspeed1 ==
  Vb : Inport  Unit=m/s
  Airspeed : Sqrt  AlgorithmType=Newton-Raphson  SaturateOnIntegerOverflow=on
  Dot Product : DotProduct  InputSameDT=on  OutDataTypeStr=Inherit: Inherit via internal rule
  Incidence : Trigonometry  Operator=atan2
  Product : Product  Inputs=*/  SaturateOnIntegerOverflow=on  OutDataTypeStr=Inherit: Same as first input
  Selector : Selector  InputPortWidth=3  IndexOptions=Index vector (dialog)  Indices=[2]  OutputSizes=1
  Selector1 : Selector  InputPortWidth=3  IndexOptions=Index vector (dialog)  Indices=[3]  OutputSizes=1
  Selector2 : Selector  InputPortWidth=3  IndexOptions=Index vector (dialog)  Indices=[1]  OutputSizes=1
  Sideslip : Trigonometry  Operator=asin
  Alpha : Outport  Unit=rad  InitialOutput=0
  Beta : Outport  Port=2  Unit=rad  InitialOutput=0
  V : Outport  Port=3  Unit=m/s  InitialOutput=0
  wires:
  Selector/1 -> Product/1
  Sideslip/1 -> Beta/1
  Vb/1 -> Dot Product/2, Dot Product/1, Selector/1, Selector2/1, Selector1/1
  Incidence/1 -> Alpha/1
  Airspeed/1 -> V/1, Product/2
  Dot Product/1 -> Airspeed/1
  Selector2/1 -> Incidence/2
  Selector1/1 -> Incidence/1
  Product/1 -> Sideslip/1

== system DatcomNew/My Digital DATCOM v1.0.3/Dynamic Contribution/Stability Angular Rates ==
  alpha beta : Inport  Unit=rad
  alphadot betadot : Inport  Port=2  Unit=rad/s
  p,q,r : Inport  Port=3  Unit=rad/s
  Demux : Demux  Outputs=2
  Direction Cosine Matrix Body to Wind : aerolibtransform2/Direction Cosine Matrix Body to Wind
      settings: SourceProductName=Aerospace Blockset  SourceProductBaseCode=AE
  Disallow CGS : UnitConfiguration  UnitSystemsStr=English,SI,SI (extended)  AllowAllUnitSystems=off
  Mux : Mux  Inputs=3
  Product : Product  RndMeth=Zero
  Product1 : Product  Multiplication=Matrix(*)  SaturateOnIntegerOverflow=on  InputSameDT=on  OutDataTypeStr=Inherit: Same as first input
  Product2 : Product  RndMeth=Zero
  SinCos : Trigonometry  Operator=sincos
  Subsystem : aerolibasang/Wind Angular Rates/Subsystem
      settings: SourceProductName=Aerospace Blockset  SourceProductBaseCode=AE
  Sum : Sum  Inputs=|++
  Unary Minus : UnaryMinus
  Unary Minus1 : UnaryMinus
  p,q,r wind : Outport  Unit=rad/s  InitialOutput=0
  wires:
  alpha beta/1 -> Direction Cosine Matrix Body to Wind/1, Subsystem/1
  Subsystem/1 -> SinCos/1
  SinCos/1 -> Product/2
  SinCos/2 -> Product2/2
  Direction Cosine Matrix Body to Wind/1 -> Product1/1
  Sum/1 -> Product1/2
  Product1/1 -> p,q,r wind/1
  Mux/1 -> Sum/1
  p,q,r/1 -> Sum/2
  alphadot betadot/1 -> Demux/1
  Demux/2 -> Product2/1, Product/1
  Demux/1 -> Unary Minus/1
  Product/1 -> Unary Minus1/1
  Product2/1 -> Mux/3
  Unary Minus1/1 -> Mux/1
  Unary Minus/1 -> Mux/2

== system DatcomNew/My Digital DATCOM v1.0.3/Static Contribution/Aerodynamic Forces and Moments ==
  Coefficients : Inport
  qbar : Inport  Port=2  Unit=Pa
  CG : Inport  Port=3  Unit=m  PortDimensions=[3, 1]
  CP : Inport  Port=4  Unit=m  PortDimensions=[3,1]
  Vb : Inport  Port=5
  S ref : Inport  Port=6  Unit=m^2  PortDimensions=1
  b ref : Inport  Port=7  Unit=m  PortDimensions=1
  cbar : Inport  Port=8  Unit=m  PortDimensions=1
  3x3 Cross Product : aerolibutil/3x3 Cross Product
      settings: SourceProductName=Aerospace Blockset  SourceProductBaseCode=AE
  CG-CP Transformation : Subsystem
  Demux1 : Demux  Outputs=[3,3]
  Force Transformation : Subsystem
  Moment Transformation : Subsystem
  Mux : Mux  Inputs=3
  Product{,1..3} (4 alike) : Product  SaturateOnIntegerOverflow=on  InputSameDT=on  OutDataTypeStr=Inherit: Same as first input
  Sum : Sum  Inputs=|+-  SaturateOnIntegerOverflow=on
  Sum1 : Sum  Inputs=++|  SaturateOnIntegerOverflow=on  InputSameDT=on  OutDataTypeStr=Inherit: Same as first input
  Vb2 : InportShadow  Port=5
  coefAdjust : Gain  Gain="[-1  1 -1]"
  Forces : Outport  Unit=N
  Moments : Outport  Port=2  Unit=N*m
  wires:
  Vb2/1 -> Moment Transformation/1(Vb)
  Sum1/1 -> Moment Transformation/2(Property-In-Stability (PIS))
  S ref/1 -> Product2/2
  Mux/1 -> Product1/1
  b ref/1 -> Mux/3, Mux/1
  cbar/1 -> Mux/2
  3x3 Cross Product/1 -> Sum1/1
  Product1/1 -> Product3/2
  Coefficients/1 -> Demux1/1
  Demux1/2 -> Product3/1
  qbar/1 -> Product2/1
  Product2/1 -> Product1/2, Product/1
  Product3/1 -> Sum1/2
  Demux1/1 -> coefAdjust/1
  Product/1 -> Force Transformation/2(Property-In-Stability (PIS)), 3x3 Cross Product/1
  Force Transformation/1(Property-In-Body (PIB)) -> Forces/1
  Moment Transformation/1(Property-In-Body (PIB)) -> Moments/1
  coefAdjust/1 -> Product/2
  CG/1 -> Sum/1
  CP/1 -> Sum/2
  Sum/1 -> CG-CP Transformation/2(Property-In-Stability (PIS))
  CG-CP Transformation/1(Property-In-Body (PIB)) -> 3x3 Cross Product/2
  Vb/1 -> Force Transformation/1(Vb), CG-CP Transformation/1(Vb)

== system DatcomNew/My Digital DATCOM v1.0.1/Deflection/Aerodynamic Forces and Moments/CG-CP Transformation ==
  Vb : Inport
  Property-In-Stability (PIS) : Inport  Port=2
  Body2Stability : Subsystem
  "Incidence, Sideslip, & Airspeed" : Subsystem
      mask Display:
      | port_label('input',1,'V_b','texmode','on');
      | port_label('output',1,'\alpha','texmode','on');
      | port_label('output',2,'\beta','texmode','on');
      | port_label('output',3,'V','texmode','on');
  Product : Product  Multiplication=Matrix(*)  RndMeth=Zero
  Terminator : Terminator
  Terminator1 : Terminator
  Transpose : Math  Operator=transpose  SaturateOnIntegerOverflow=on
  Property-In-Body (PIB) : Outport
  wires:
  "Incidence, Sideslip, & Airspeed"/3(V) -> Terminator1/1
  "Incidence, Sideslip, & Airspeed"/2(Beta) -> Terminator/1
  Vb/1 -> "Incidence, Sideslip, & Airspeed"/1(Vb)
  Transpose/1 -> Product/1  "Stability2Body"
  Body2Stability/1(Ts/b) -> Transpose/1
  "Incidence, Sideslip, & Airspeed"/1(Alpha) -> Body2Stability/1(alpha)
  Property-In-Stability (PIS)/1 -> Product/2
  Product/1 -> Property-In-Body (PIB)/1

== system DatcomNew/My Digital DATCOM v1.0.1/Deflection/Aerodynamic Forces and Moments/Force Transformation ==
  Vb : Inport
  Property-In-Stability (PIS) : Inport  Port=2
  Body2Stability : Subsystem
  "Incidence, Sideslip, & Airspeed" : Subsystem
      mask Display:
      | port_label('input',1,'V_b','texmode','on');
      | port_label('output',1,'\alpha','texmode','on');
      | port_label('output',2,'\beta','texmode','on');
      | port_label('output',3,'V','texmode','on');
  Product : Product  Multiplication=Matrix(*)  RndMeth=Zero
  Terminator : Terminator
  Terminator1 : Terminator
  Transpose : Math  Operator=transpose  SaturateOnIntegerOverflow=on
  Property-In-Body (PIB) : Outport
  wires:
  "Incidence, Sideslip, & Airspeed"/3(V) -> Terminator1/1
  "Incidence, Sideslip, & Airspeed"/2(Beta) -> Terminator/1
  Vb/1 -> "Incidence, Sideslip, & Airspeed"/1(Vb)
  Transpose/1 -> Product/1  "Stability2Body"
  Body2Stability/1(Ts/b) -> Transpose/1
  "Incidence, Sideslip, & Airspeed"/1(Alpha) -> Body2Stability/1(alpha)
  Property-In-Stability (PIS)/1 -> Product/2
  Product/1 -> Property-In-Body (PIB)/1

== system DatcomNew/My Digital DATCOM v1.0.1/Deflection/Aerodynamic Forces and Moments/Moment Transformation ==
  Vb : Inport
  Property-In-Stability (PIS) : Inport  Port=2
  Body2Stability : Subsystem
  "Incidence, Sideslip, & Airspeed" : Subsystem
      mask Display:
      | port_label('input',1,'V_b','texmode','on');
      | port_label('output',1,'\alpha','texmode','on');
      | port_label('output',2,'\beta','texmode','on');
      | port_label('output',3,'V','texmode','on');
  Product : Product  Multiplication=Matrix(*)  RndMeth=Zero
  Terminator : Terminator
  Terminator1 : Terminator
  Transpose : Math  Operator=transpose  SaturateOnIntegerOverflow=on
  Property-In-Body (PIB) : Outport
  wires:
  Product/1 -> Property-In-Body (PIB)/1
  Property-In-Stability (PIS)/1 -> Product/2
  "Incidence, Sideslip, & Airspeed"/1(Alpha) -> Body2Stability/1(alpha)
  Body2Stability/1(Ts/b) -> Transpose/1
  Transpose/1 -> Product/1  "Stability2Body"
  Vb/1 -> "Incidence, Sideslip, & Airspeed"/1(Vb)
  "Incidence, Sideslip, & Airspeed"/2(Beta) -> Terminator/1
  "Incidence, Sideslip, & Airspeed"/3(V) -> Terminator1/1

== system DatcomNew/My Digital DATCOM v1.0.1/Deflection/Delta Coefficients/Aileron Deflaction ==
  bus : Inport
  Bus Selector : BusSelector  OutputSignals=idxa,fa,idxm,fm,idxh,fh,idxd_a,fd_a
  Bus Selector1 : BusSelector  OutputSignals=idxa,fa,idxm,fm,idxh,fh,idxd_a,fd_a
  Constant{1,4..6} (4 alike) : Constant  Value=0
  DCl : Interpolation_n-D  NumberOfTableDimensions=4  Table=permute(datcom.dcl_de,[1 2 3 4])  RemoveProtectionIndex=on
      settings: InputPortMap=u0,u1,u2,u3,u4,u5,u6,u7
  DCn : Interpolation_n-D  NumberOfTableDimensions=4  Table=permute(datcom.dcdi_de,[1 2 3 4])  RemoveProtectionIndex=on
      settings: InputPortMap=u0,u1,u2,u3,u4,u5,u6,u7
  Mux1 : Mux  Inputs=6
  delCoeff_a : Outport
  wires:
  Bus Selector/4 -> DCn/4  "<fm>"
  Bus Selector/5 -> DCn/5  "<idxh>"
  Bus Selector/2 -> DCn/2  "<fa>"
  Bus Selector/1 -> DCn/1  "<idxa>"
  Bus Selector/8 -> DCn/8  "<fd_a>"
  Bus Selector/6 -> DCn/6  "<fh>"
  Mux1/1 -> delCoeff_a/1
  Bus Selector1/1 -> DCl/1  "<idxa>"
  Bus Selector1/5 -> DCl/5  "<idxh>"
  Bus Selector1/2 -> DCl/2  "<fa>"
  Bus Selector1/8 -> DCl/8  "<fd_a>"
  Bus Selector1/6 -> DCl/6  "<fh>"
  Bus Selector1/4 -> DCl/4  "<fm>"
  bus/1 -> Bus Selector1/1, Bus Selector/1
  Constant4/1 -> Mux1/5  "Cm_a"
  Constant5/1 -> Mux1/3  "CL_e"
  Constant1/1 -> Mux1/2  "CY_a"
  Constant6/1 -> Mux1/1  "CD_a"
  DCn/1 -> Mux1/6  "Cn_a"
  DCl/1 -> Mux1/4  "Cl_a"
  Bus Selector1/3 -> DCl/3  "<idxm>"
  Bus Selector1/7 -> DCl/7  "<idxd_a>"
  Bus Selector/3 -> DCn/3  "<idxm>"
  Bus Selector/7 -> DCn/7  "<idxd_a>"

== system DatcomNew/My Digital DATCOM v1.0.1/Deflection/Delta Coefficients/Elevator Deflaction ==
  bus : Inport
  Bus Selector : BusSelector  OutputSignals=idxa,fa,idxm,fm,idxh,fh,idxd_e,fd_e
  Bus Selector1 : BusSelector  OutputSignals=idxa,fa,idxm,fm,idxh,fh,idxd_e,fd_e
  Bus Selector2 : BusSelector  OutputSignals=idxa,fa,idxm,fm,idxh,fh,idxd_e,fd_e
  Constant1 : Constant  Value=0
  Constant2 : Constant  Value=0
  Constant3 : Constant  Value=0
  DCDI : Interpolation_n-D  NumberOfTableDimensions=4  Table=permute(datcom.dcdi_de,[1 2 3 4])  RemoveProtectionIndex=on
      settings: InputPortMap=u0,u1,u2,u3,u4,u5,u6,u7
  DCL : Interpolation_n-D  NumberOfTableDimensions=4  Table=permute(datcom.dcl_de,[1 2 3 4])  RemoveProtectionIndex=on
      settings: InputPortMap=u0,u1,u2,u3,u4,u5,u6,u7
  DCm : Interpolation_n-D  NumberOfTableDimensions=4  Table=permute(datcom.dcm_de,[1 2 3 4])  RemoveProtectionIndex=on
      settings: InputPortMap=u0,u1,u2,u3,u4,u5,u6,u7
  Mux1 : Mux  Inputs=6
  delCoeff_e : Outport
  wires:
  bus/1 -> Bus Selector2/1, Bus Selector1/1, Bus Selector/1
  Bus Selector1/4 -> DCL/4  "<fm>"
  Bus Selector1/6 -> DCL/6  "<fh>"
  Bus Selector1/8 -> DCL/8  "<fd_e>"
  Bus Selector2/6 -> DCm/6  "<fh>"
  Bus Selector2/2 -> DCm/2  "<fa>"
  Bus Selector2/4 -> DCm/4  "<fm>"
  Bus Selector2/5 -> DCm/5  "<idxh>"
  Bus Selector2/8 -> DCm/8  "<fd_e>"
  Bus Selector2/1 -> DCm/1  "<idxa>"
  Bus Selector1/2 -> DCL/2  "<fa>"
  Bus Selector1/5 -> DCL/5  "<idxh>"
  Bus Selector1/1 -> DCL/1  "<idxa>"
  Mux1/1 -> delCoeff_e/1
  Bus Selector/6 -> DCDI/6  "<fh>"
  Bus Selector/8 -> DCDI/8  "<fd_e>"
  Bus Selector/1 -> DCDI/1  "<idxa>"
  Bus Selector/2 -> DCDI/2  "<fa>"
  Bus Selector/5 -> DCDI/5  "<idxh>"
  Bus Selector/4 -> DCDI/4  "<fm>"
  DCm/1 -> Mux1/5  "Cm_e"
  DCL/1 -> Mux1/3  "CL_e"
  Constant1/1 -> Mux1/2  "CY_e"
  DCDI/1 -> Mux1/1  "CD_e"
  Constant3/1 -> Mux1/6  "Cn_e"
  Constant2/1 -> Mux1/4  "Cl_e"
  Bus Selector/7 -> DCDI/7  "<idxd_e>"
  Bus Selector/3 -> DCDI/3  "<idxm>"
  Bus Selector1/3 -> DCL/3  "<idxm>"
  Bus Selector1/7 -> DCL/7  "<idxd_e>"
  Bus Selector2/7 -> DCm/7  "<idxd_e>"
  Bus Selector2/3 -> DCm/3  "<idxm>"

== system DatcomNew/My Digital DATCOM v1.0.1/Deflection/Delta Coefficients/Flap Deflaction ==
  bus : Inport
  Bus Selector : BusSelector  OutputSignals=idxa,fa,idxm,fm,idxh,fh,idxd_f,fd_f
  Bus Selector1 : BusSelector  OutputSignals=idxa,fa,idxm,fm,idxh,fh,idxd_f,fd_f
  Bus Selector4 : BusSelector  OutputSignals=idxa,fa,idxm,fm,idxh,fh,idxd_f,fd_f
  Constant1 : Constant  Value=0
  Constant2 : Constant  Value=0
  Constant3 : Constant  Value=0
  DCDI : Interpolation_n-D  NumberOfTableDimensions=4  Table=permute(datcom.dcdi_df,[1 2 3 4])  RemoveProtectionIndex=on
      settings: InputPortMap=u0,u1,u2,u3,u4,u5,u6,u7
  DCL : Interpolation_n-D  NumberOfTableDimensions=4  Table=permute(datcom.dcl_df,[1 2 3 4])  RemoveProtectionIndex=on
      settings: InputPortMap=u0,u1,u2,u3,u4,u5,u6,u7
  DCm : Interpolation_n-D  NumberOfTableDimensions=4  Table=permute(datcom.dcm_df,[1 2 3 4])  RemoveProtectionIndex=on
      settings: InputPortMap=u0,u1,u2,u3,u4,u5,u6,u7
  Mux1 : Mux  Inputs=6
  delCoeff_f : Outport
  wires:
  Bus Selector/4 -> DCDI/4  "<fm>"
  Bus Selector/5 -> DCDI/5  "<idxh>"
  Bus Selector/2 -> DCDI/2  "<fa>"
  Bus Selector/1 -> DCDI/1  "<idxa>"
  Bus Selector/8 -> DCDI/8  "<fd_f>"
  Bus Selector/6 -> DCDI/6  "<fh>"
  Mux1/1 -> delCoeff_f/1
  DCm/1 -> Mux1/5  "Cm_f"
  Bus Selector1/1 -> DCL/1  "<idxa>"
  Bus Selector1/5 -> DCL/5  "<idxh>"
  Bus Selector1/2 -> DCL/2  "<fa>"
  Bus Selector4/1 -> DCm/1  "<idxa>"
  Bus Selector4/8 -> DCm/8  "<fd_f>"
  Bus Selector4/5 -> DCm/5  "<idxh>"
  Bus Selector4/4 -> DCm/4  "<fm>"
  Bus Selector4/2 -> DCm/2  "<fa>"
  Bus Selector4/6 -> DCm/6  "<fh>"
  Bus Selector1/8 -> DCL/8  "<fd_f>"
  DCL/1 -> Mux1/3  "CL_f"
  Constant1/1 -> Mux1/2  "CY_f"
  DCDI/1 -> Mux1/1  "CD_f"
  Bus Selector1/6 -> DCL/6  "<fh>"
  Bus Selector1/4 -> DCL/4  "<fm>"
  bus/1 -> Bus Selector/1, Bus Selector4/1, Bus Selector1/1
  Constant3/1 -> Mux1/6  "Cn_f"
  Constant2/1 -> Mux1/4  "Cl_f"
  Bus Selector/3 -> DCDI/3  "<idxm>"
  Bus Selector/7 -> DCDI/7  "<idxd_f>"
  Bus Selector1/3 -> DCL/3  "<idxm>"
  Bus Selector1/7 -> DCL/7  "<idxd_f>"
  Bus Selector4/7 -> DCm/7  "<idxd_f>"
  Bus Selector4/3 -> DCm/3  "<idxm>"

== system DatcomNew/My Digital DATCOM v1.0.1/Dynamic Contribution/Aerodynamic Forces and Moments Stability Axis/CG-CP Transformation ==
  Vb : Inport
  Property-In-Stability (PIS) : Inport  Port=2
  Body2Stability : Subsystem
  "Incidence, Sideslip, & Airspeed" : Subsystem
      mask Display:
      | port_label('input',1,'V_b','texmode','on');
      | port_label('output',1,'\alpha','texmode','on');
      | port_label('output',2,'\beta','texmode','on');
      | port_label('output',3,'V','texmode','on');
  Product : Product  Multiplication=Matrix(*)  RndMeth=Zero
  Terminator : Terminator
  Terminator1 : Terminator
  Transpose : Math  Operator=transpose  SaturateOnIntegerOverflow=on
  Property-In-Body (PIB) : Outport
  wires:
  "Incidence, Sideslip, & Airspeed"/3(V) -> Terminator1/1
  "Incidence, Sideslip, & Airspeed"/2(Beta) -> Terminator/1
  Vb/1 -> "Incidence, Sideslip, & Airspeed"/1(Vb)
  Transpose/1 -> Product/1  "Stability2Body"
  Body2Stability/1(Ts/b) -> Transpose/1
  "Incidence, Sideslip, & Airspeed"/1(Alpha) -> Body2Stability/1(alpha)
  Property-In-Stability (PIS)/1 -> Product/2
  Product/1 -> Property-In-Body (PIB)/1

== system DatcomNew/My Digital DATCOM v1.0.1/Dynamic Contribution/Aerodynamic Forces and Moments Stability Axis/Force Transformation ==
  Vb : Inport
  Property-In-Stability (PIS) : Inport  Port=2
  Body2Stability : Subsystem
  "Incidence, Sideslip, & Airspeed" : Subsystem
      mask Display:
      | port_label('input',1,'V_b','texmode','on');
      | port_label('output',1,'\alpha','texmode','on');
      | port_label('output',2,'\beta','texmode','on');
      | port_label('output',3,'V','texmode','on');
  Product : Product  Multiplication=Matrix(*)  RndMeth=Zero
  Terminator : Terminator
  Terminator1 : Terminator
  Transpose : Math  Operator=transpose  SaturateOnIntegerOverflow=on
  Property-In-Body (PIB) : Outport
  wires:
  "Incidence, Sideslip, & Airspeed"/3(V) -> Terminator1/1
  "Incidence, Sideslip, & Airspeed"/2(Beta) -> Terminator/1
  Vb/1 -> "Incidence, Sideslip, & Airspeed"/1(Vb)
  Transpose/1 -> Product/1  "Stability2Body"
  Body2Stability/1(Ts/b) -> Transpose/1
  "Incidence, Sideslip, & Airspeed"/1(Alpha) -> Body2Stability/1(alpha)
  Property-In-Stability (PIS)/1 -> Product/2
  Product/1 -> Property-In-Body (PIB)/1

== system DatcomNew/My Digital DATCOM v1.0.1/Dynamic Contribution/Aerodynamic Forces and Moments Stability Axis/Moment Transformation ==
  Vb : Inport
  Property-In-Stability (PIS) : Inport  Port=2
  Body2Stability : Subsystem
  "Incidence, Sideslip, & Airspeed" : Subsystem
      mask Display:
      | port_label('input',1,'V_b','texmode','on');
      | port_label('output',1,'\alpha','texmode','on');
      | port_label('output',2,'\beta','texmode','on');
      | port_label('output',3,'V','texmode','on');
  Product : Product  Multiplication=Matrix(*)  RndMeth=Zero
  Terminator : Terminator
  Terminator1 : Terminator
  Transpose : Math  Operator=transpose  SaturateOnIntegerOverflow=on
  Property-In-Body (PIB) : Outport
  wires:
  Product/1 -> Property-In-Body (PIB)/1
  Property-In-Stability (PIS)/1 -> Product/2
  "Incidence, Sideslip, & Airspeed"/1(Alpha) -> Body2Stability/1(alpha)
  Body2Stability/1(Ts/b) -> Transpose/1
  Transpose/1 -> Product/1  "Stability2Body"
  Vb/1 -> "Incidence, Sideslip, & Airspeed"/1(Vb)
  "Incidence, Sideslip, & Airspeed"/2(Beta) -> Terminator/1
  "Incidence, Sideslip, & Airspeed"/3(V) -> Terminator1/1

== system DatcomNew/My Digital DATCOM v1.0.1/Static Contribution/Aerodynamic Forces and Moments/CG-CP Transformation ==
  Vb : Inport
  Property-In-Stability (PIS) : Inport  Port=2
  Body2Stability : Subsystem
  "Incidence, Sideslip, & Airspeed" : Subsystem
      mask Display:
      | port_label('input',1,'V_b','texmode','on');
      | port_label('output',1,'\alpha','texmode','on');
      | port_label('output',2,'\beta','texmode','on');
      | port_label('output',3,'V','texmode','on');
  Product : Product  Multiplication=Matrix(*)  RndMeth=Zero
  Terminator : Terminator
  Terminator1 : Terminator
  Transpose : Math  Operator=transpose  SaturateOnIntegerOverflow=on
  Property-In-Body (PIB) : Outport
  wires:
  "Incidence, Sideslip, & Airspeed"/3(V) -> Terminator1/1
  "Incidence, Sideslip, & Airspeed"/2(Beta) -> Terminator/1
  Vb/1 -> "Incidence, Sideslip, & Airspeed"/1(Vb)
  Transpose/1 -> Product/1  "Stability2Body"
  Body2Stability/1(Ts/b) -> Transpose/1
  "Incidence, Sideslip, & Airspeed"/1(Alpha) -> Body2Stability/1(alpha)
  Property-In-Stability (PIS)/1 -> Product/2
  Product/1 -> Property-In-Body (PIB)/1

== system DatcomNew/My Digital DATCOM v1.0.1/Static Contribution/Aerodynamic Forces and Moments/Force Transformation ==
  Vb : Inport
  Property-In-Stability (PIS) : Inport  Port=2
  Body2Stability : Subsystem
  "Incidence, Sideslip, & Airspeed" : Subsystem
      mask Display:
      | port_label('input',1,'V_b','texmode','on');
      | port_label('output',1,'\alpha','texmode','on');
      | port_label('output',2,'\beta','texmode','on');
      | port_label('output',3,'V','texmode','on');
  Product : Product  Multiplication=Matrix(*)  RndMeth=Zero
  Terminator : Terminator
  Terminator1 : Terminator
  Transpose : Math  Operator=transpose  SaturateOnIntegerOverflow=on
  Property-In-Body (PIB) : Outport
  wires:
  "Incidence, Sideslip, & Airspeed"/3(V) -> Terminator1/1
  "Incidence, Sideslip, & Airspeed"/2(Beta) -> Terminator/1
  Vb/1 -> "Incidence, Sideslip, & Airspeed"/1(Vb)
  Transpose/1 -> Product/1  "Stability2Body"
  Body2Stability/1(Ts/b) -> Transpose/1
  "Incidence, Sideslip, & Airspeed"/1(Alpha) -> Body2Stability/1(alpha)
  Property-In-Stability (PIS)/1 -> Product/2
  Product/1 -> Property-In-Body (PIB)/1

== system DatcomNew/My Digital DATCOM v1.0.1/Static Contribution/Aerodynamic Forces and Moments/Moment Transformation ==
  Vb : Inport
  Property-In-Stability (PIS) : Inport  Port=2
  Body2Stability : Subsystem
  "Incidence, Sideslip, & Airspeed" : Subsystem
      mask Display:
      | port_label('input',1,'V_b','texmode','on');
      | port_label('output',1,'\alpha','texmode','on');
      | port_label('output',2,'\beta','texmode','on');
      | port_label('output',3,'V','texmode','on');
  Product : Product  Multiplication=Matrix(*)  RndMeth=Zero
  Terminator : Terminator
  Terminator1 : Terminator
  Transpose : Math  Operator=transpose  SaturateOnIntegerOverflow=on
  Property-In-Body (PIB) : Outport
  wires:
  Product/1 -> Property-In-Body (PIB)/1
  Property-In-Stability (PIS)/1 -> Product/2
  "Incidence, Sideslip, & Airspeed"/1(Alpha) -> Body2Stability/1(alpha)
  Body2Stability/1(Ts/b) -> Transpose/1
  Transpose/1 -> Product/1  "Stability2Body"
  Vb/1 -> "Incidence, Sideslip, & Airspeed"/1(Vb)
  "Incidence, Sideslip, & Airspeed"/2(Beta) -> Terminator/1
  "Incidence, Sideslip, & Airspeed"/3(V) -> Terminator1/1

== system DatcomNew/My Digital DATCOM v1.0.2/Deflection/Aerodynamic Forces and Moments/CG-CP Transformation ==
  Vb : Inport
  Property-In-Stability (PIS) : Inport  Port=2
  Body2Stability : Subsystem
  "Incidence, Sideslip, & Airspeed" : Subsystem
      mask Display:
      | port_label('input',1,'V_b','texmode','on');
      | port_label('output',1,'\alpha','texmode','on');
      | port_label('output',2,'\beta','texmode','on');
      | port_label('output',3,'V','texmode','on');
  Product : Product  Multiplication=Matrix(*)  RndMeth=Zero
  Terminator : Terminator
  Terminator1 : Terminator
  Transpose : Math  Operator=transpose  SaturateOnIntegerOverflow=on
  Property-In-Body (PIB) : Outport
  wires:
  Product/1 -> Property-In-Body (PIB)/1
  Property-In-Stability (PIS)/1 -> Product/2
  "Incidence, Sideslip, & Airspeed"/1(Alpha) -> Body2Stability/1(alpha)
  Body2Stability/1(Ts/b) -> Transpose/1
  Transpose/1 -> Product/1  "Stability2Body"
  Vb/1 -> "Incidence, Sideslip, & Airspeed"/1(Vb)
  "Incidence, Sideslip, & Airspeed"/2(Beta) -> Terminator/1
  "Incidence, Sideslip, & Airspeed"/3(V) -> Terminator1/1
